simulink model "3.Clark_Park"  (R2022b)
settings: Solver=ode45  StartTime=0.0  StopTime=0.03  RelTol=1e-3
libraries: spsAlphaBetaZerotodq0Lib x1, spsabctoAlphaBetaZeroLib x1
settings Model: Creator=Mushrif  LastModifiedBy=Mushrif

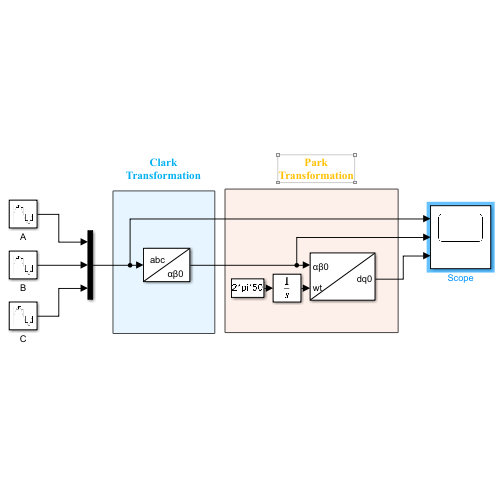
[thumbnail: Simulink's stored preview of the top-level diagram]
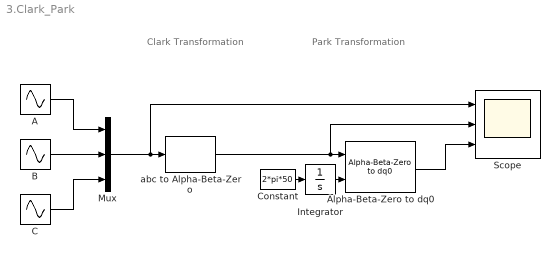
== system 3.Clark_Park ==
  note: Clark
      | Transformation
  note: Park
      | Transformation
  A : Sin  Frequency=2*pi*50  SampleTime=1e-8
  Alpha-Beta-Zero to dq0 : spsAlphaBetaZerotodq0Lib/Alpha-Beta-Zero to dq0  Alignment=90 degrees behind phase A axis
  B : Sin  Frequency=2*pi*50  Phase=-120*pi/180  SampleTime=1e-8
  C : Sin  Frequency=2*pi*50  Phase=120*pi/180  SampleTime=1e-8
  Constant : Constant  Value=2*pi*50
  Integrator : Integrator
  Mux : Mux  Inputs=3
  Scope : Scope  NumInputPorts=3
  abc to Alpha-Beta-Zero : spsabctoAlphaBetaZeroLib/abc to Alpha-Beta-Zero
  wires:
  B/1 -> Mux/2
  A/1 -> Mux/1
  C/1 -> Mux/3
  Mux/1 -> Scope/1, abc to Alpha-Beta-Zero/1
  abc to Alpha-Beta-Zero/1 -> Scope/2, Alpha-Beta-Zero to dq0/1
  Constant/1 -> Integrator/1
  Integrator/1 -> Alpha-Beta-Zero to dq0/2
  Alpha-Beta-Zero to dq0/1 -> Scope/3
